simulink model "model1"  (Simulink 7.6)
settings: Solver=FixedStepDiscrete  StartTime=0.0  StopTime=10  FixedStep=1  RelTol=1e-3
libraries: simulink x6
settings Model: Creator=jordan  LastModifiedBy=jordan
settings OptimizationCC: BlockReduction=off  ConditionallyExecuteInputs=off

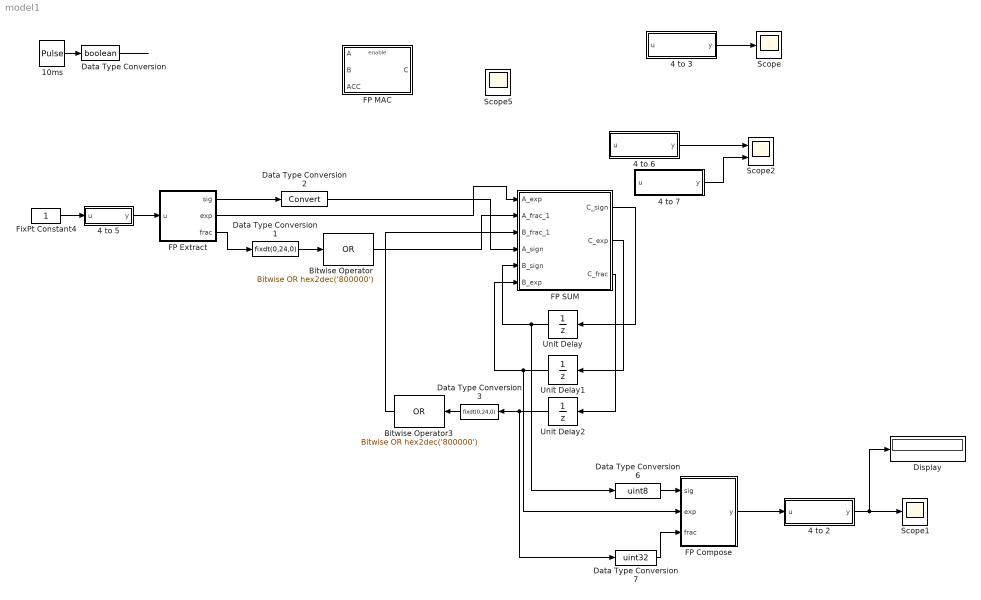
== system model1 ==
  10ms : DiscretePulseGenerator  Period=100
  4 to 2 : Stateflow chart  TreatAsAtomicUnit=on
  4 to 3 : Stateflow chart  TreatAsAtomicUnit=on
  4 to 5 : Stateflow chart  TreatAsAtomicUnit=on
  4 to 6 : Stateflow chart  TreatAsAtomicUnit=on
  4 to 7 : Stateflow chart  TreatAsAtomicUnit=on
  Bitwise Operator : simulink/Logic and Bit Operations/Bitwise Operator  logicop=OR  UseBitMask=on  BitMask=hex2dec('800000')  BitMaskRealWorld=Stored Integer
  Bitwise Operator3 : simulink/Logic and Bit Operations/Bitwise Operator  logicop=OR  UseBitMask=on  BitMask=hex2dec('800000')  BitMaskRealWorld=Stored Integer
  Data Type Conversion : DataTypeConversion  OutDataTypeStr=boolean
  Data Type Conversion1 : DataTypeConversion  OutDataTypeStr=fixdt(0,24,0)  RndMeth=Nearest
  Data Type Conversion2 : DataTypeConversion  RndMeth=Nearest
  Data Type Conversion3 : DataTypeConversion  OutDataTypeStr=fixdt(0,24,0)  RndMeth=Nearest
  Data Type Conversion6 : DataTypeConversion  OutDataTypeStr=uint8  RndMeth=Nearest
  Data Type Conversion7 : DataTypeConversion  OutDataTypeStr=uint32  RndMeth=Nearest
  Display : Display
  FP Compose : Stateflow chart  TreatAsAtomicUnit=on
  FP Extract : Stateflow chart  TreatAsAtomicUnit=on
  FP MAC : Subsystem
  FP SUM : Subsystem
  FixPt Constant4 : Constant  DisableCoverage=on  OutDataTypeStr=single  LockScale=on
  Scope : Scope
      settings: TimeRange=20.20725388601036  YMin=0  YMax=100  MaxDataPoints=50000
  Scope1 : Scope
      settings: SaveName=ScopeData3  MaxDataPoints=50000
  Scope2 : Scope  NumInputPorts=2
      settings: YMin=-5~-5  YMax=5~5  SaveName=ScopeData4  MaxDataPoints=50000
  Scope5 : Scope
      settings: SaveName=ScopeData11  MaxDataPoints=50000
  Unit Delay : UnitDelay  SampleTime=-1
  Unit Delay1 : UnitDelay  SampleTime=-1
  Unit Delay2 : UnitDelay  SampleTime=-1
  wires:
  10ms/1 -> Data Type Conversion/1
  Data Type Conversion/1 -> ?
  4 to 2/1(y) -> Scope1/1, Display/1
  4 to 6/1(y) -> Scope2/1
  4 to 7/1(y) -> Scope2/2
  4 to 3/1(y) -> Scope/1
  FP SUM/1(C_sign) -> Unit Delay/1
  FP SUM/2(C_exp) -> Unit Delay1/1
  FP SUM/3(C_frac) -> Unit Delay2/1
  Unit Delay/1 -> FP SUM/5(B_sign), Data Type Conversion6/1
  Unit Delay1/1 -> FP SUM/6(B_exp), FP Compose/2(exp)
  Unit Delay2/1 -> Data Type Conversion3/1, Data Type Conversion7/1
  Data Type Conversion3/1 -> Bitwise Operator3/1
  Bitwise Operator3/1 -> FP SUM/3(B_frac_1)
  FP Extract/1(sig) -> Data Type Conversion2/1
  FP Extract/2(exp) -> FP SUM/1(A_exp)
  Data Type Conversion1/1 -> Bitwise Operator/1
  FP Extract/3(frac) -> Data Type Conversion1/1
  Bitwise Operator/1 -> FP SUM/2(A_frac_1)
  Data Type Conversion6/1 -> FP Compose/1(sig)
  Data Type Conversion7/1 -> FP Compose/3(frac)
  FP Compose/1(y) -> 4 to 2/1(u)
  FixPt Constant4/1 -> 4 to 5/1(u)
  4 to 5/1(y) -> FP Extract/1(u)
  Data Type Conversion2/1 -> FP SUM/4(A_sign)

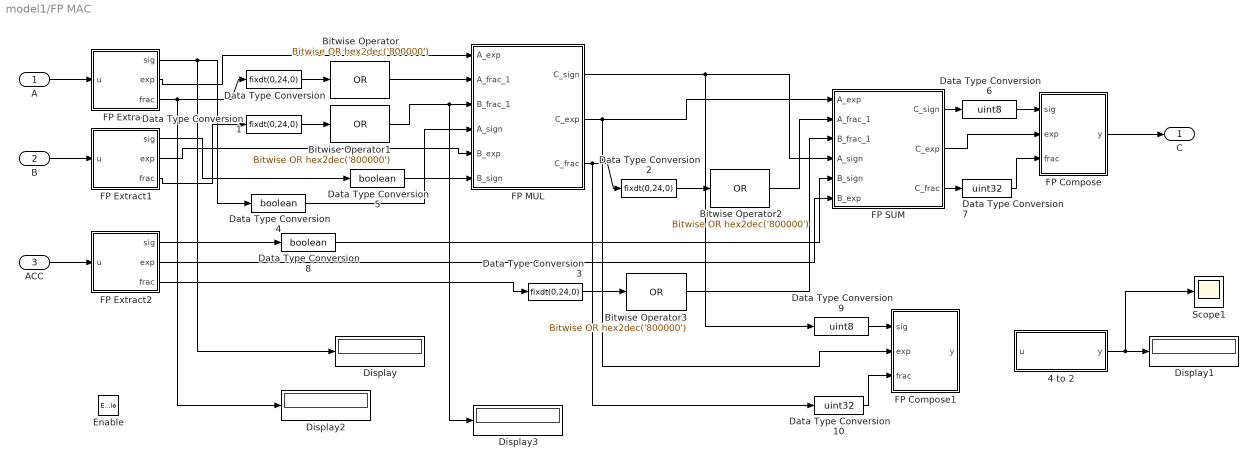
== system model1/FP MAC ==
  A : Inport
  B : Inport  Port=2
  ACC : Inport  Port=3
  Enable : EnablePort
  4 to 2 : Stateflow chart  TreatAsAtomicUnit=on
  Bitwise Operator{,1..3} (4 alike) : simulink/Logic and Bit Operations/Bitwise Operator  logicop=OR  UseBitMask=on  BitMask=hex2dec('800000')  BitMaskRealWorld=Stored Integer
  Data Type Conversion{,1..3} (4 alike) : DataTypeConversion  OutDataTypeStr=fixdt(0,24,0)  RndMeth=Nearest
  Data Type Conversion10 : DataTypeConversion  OutDataTypeStr=uint32  RndMeth=Nearest
  Data Type Conversion4 : DataTypeConversion  OutDataTypeStr=boolean  RndMeth=Nearest
  Data Type Conversion5 : DataTypeConversion  OutDataTypeStr=boolean  RndMeth=Nearest
  Data Type Conversion6 : DataTypeConversion  OutDataTypeStr=uint8  RndMeth=Nearest
  Data Type Conversion7 : DataTypeConversion  OutDataTypeStr=uint32  RndMeth=Nearest
  Data Type Conversion8 : DataTypeConversion  OutDataTypeStr=boolean  RndMeth=Nearest
  Data Type Conversion9 : DataTypeConversion  OutDataTypeStr=uint8  RndMeth=Nearest
  Display{,1..3} (4 alike) : Display
      Display3 settings: Format=hex (Stored Integer)
  FP Compose : Stateflow chart  TreatAsAtomicUnit=on
  FP Compose1 : Stateflow chart  TreatAsAtomicUnit=on
  FP Extract : Stateflow chart  TreatAsAtomicUnit=on
  FP Extract1 : Stateflow chart  TreatAsAtomicUnit=on
  FP Extract2 : Stateflow chart  TreatAsAtomicUnit=on
  FP MUL : Subsystem
  FP SUM : Subsystem
  Scope1 : Scope
      settings: SaveName=ScopeData9  MaxDataPoints=50000
  C : Outport  InitialOutput=0
  wires:
  A/1 -> FP Extract/1(u)
  B/1 -> FP Extract1/1(u)
  ACC/1 -> FP Extract2/1(u)
  FP Extract/1(sig) -> Data Type Conversion4/1, Display/1
  FP Extract1/1(sig) -> Data Type Conversion5/1
  FP Extract/2(exp) -> FP MUL/1(A_exp)
  FP Extract1/2(exp) -> FP MUL/5(B_exp)
  FP Extract/3(frac) -> Data Type Conversion/1, Display2/1
  FP Extract1/3(frac) -> Data Type Conversion1/1
  Data Type Conversion/1 -> Bitwise Operator/1
  Bitwise Operator/1 -> FP MUL/2(A_frac_1)
  Data Type Conversion1/1 -> Bitwise Operator1/1
  Bitwise Operator1/1 -> FP MUL/3(B_frac_1), Display3/1
  FP MUL/1(C_sign) -> FP SUM/4(A_sign), Data Type Conversion9/1
  FP MUL/2(C_exp) -> FP SUM/1(A_exp), FP Compose1/2(exp)
  FP MUL/3(C_frac) -> Data Type Conversion2/1, Data Type Conversion10/1
  Data Type Conversion2/1 -> Bitwise Operator2/1
  Bitwise Operator2/1 -> FP SUM/2(A_frac_1)
  FP Extract2/1(sig) -> Data Type Conversion8/1
  FP Extract2/2(exp) -> FP SUM/6(B_exp)
  FP Extract2/3(frac) -> Data Type Conversion3/1
  Data Type Conversion3/1 -> Bitwise Operator3/1
  Bitwise Operator3/1 -> FP SUM/3(B_frac_1)
  Data Type Conversion4/1 -> FP MUL/4(A_sign)
  Data Type Conversion5/1 -> FP MUL/6(B_sign)
  FP SUM/1(C_sign) -> Data Type Conversion6/1
  FP SUM/2(C_exp) -> FP Compose/2(exp)
  FP SUM/3(C_frac) -> Data Type Conversion7/1
  FP Compose/1(y) -> C/1
  Data Type Conversion6/1 -> FP Compose/1(sig)
  Data Type Conversion7/1 -> FP Compose/3(frac)
  Data Type Conversion8/1 -> FP SUM/5(B_sign)
  Data Type Conversion9/1 -> FP Compose1/1(sig)
  Data Type Conversion10/1 -> FP Compose1/3(frac)
  4 to 2/1(y) -> Display1/1, Scope1/1

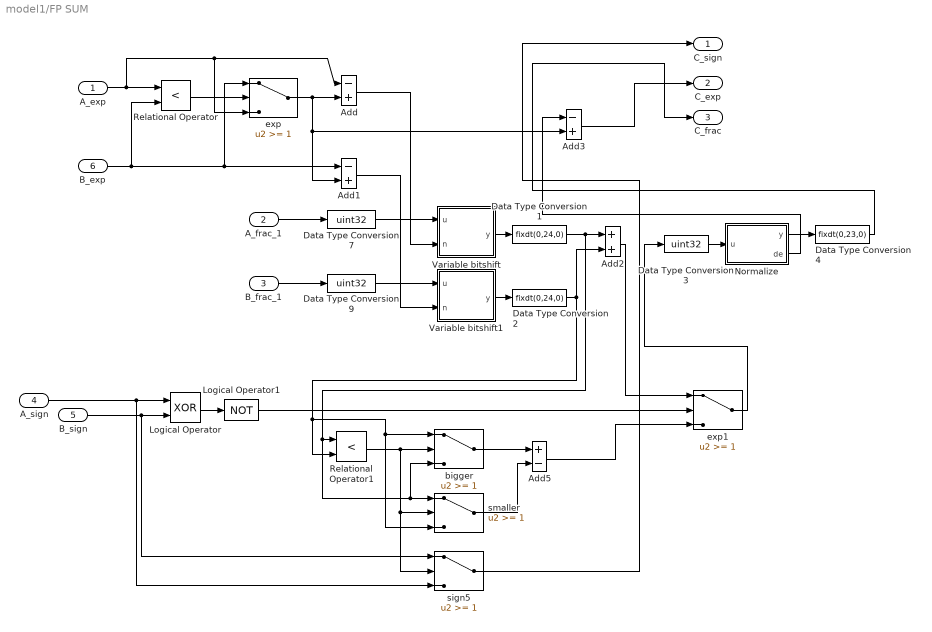
== system model1/FP SUM ==
  A_exp : Inport  OutDataTypeStr=uint8
  A_frac_1 : Inport  Port=2  OutDataTypeStr=fixdt(0,24,0)
  B_frac_1 : Inport  Port=3  OutDataTypeStr=fixdt(0,24,0)
  A_sign : Inport  Port=4  OutDataTypeStr=boolean
  B_sign : Inport  Port=5  OutDataTypeStr=boolean
  B_exp : Inport  Port=6  OutDataTypeStr=uint8
  Add : Sum  Inputs=-+  OutDataTypeStr=int8
  Add1 : Sum  Inputs=-+  OutDataTypeStr=int8
  Add2 : Sum  OutDataTypeStr=fixdt(0,25,0)  RndMeth=Nearest
  Add3 : Sum  Inputs=-+  OutDataTypeStr=uint8  SaturateOnIntegerOverflow=on
  Add5 : Sum  Inputs=+-  OutDataTypeStr=fixdt(0,25,0)  RndMeth=Nearest
  Data Type Conversion1 : DataTypeConversion  OutDataTypeStr=fixdt(0,24,0)
  Data Type Conversion2 : DataTypeConversion  OutDataTypeStr=fixdt(0,24,0)
  Data Type Conversion3 : DataTypeConversion  OutDataTypeStr=uint32
  Data Type Conversion4 : DataTypeConversion  OutDataTypeStr=fixdt(0,23,0)
  Data Type Conversion7 : DataTypeConversion  OutDataTypeStr=uint32
  Data Type Conversion9 : DataTypeConversion  OutDataTypeStr=uint32
  Logical Operator : Logic  Operator=XOR  AllPortsSameDT=off  OutDataTypeStr=boolean
  Logical Operator1 : Logic  Operator=NOT  AllPortsSameDT=off  OutDataTypeStr=boolean
  Normalize : Stateflow chart  TreatAsAtomicUnit=on
  Relational Operator : RelationalOperator  Operator=<  OutDataTypeStr=boolean
  Relational Operator1 : RelationalOperator  Operator=<  OutDataTypeStr=boolean
  Variable bitshift : Stateflow chart  TreatAsAtomicUnit=on
  Variable bitshift1 : Stateflow chart  TreatAsAtomicUnit=on
  bigger : Switch  Threshold=1
  exp : Switch  Threshold=1
  exp1 : Switch  Threshold=1
  sign5 : Switch  Threshold=1
  smaller : Switch  Threshold=1
  C_sign : Outport  OutDataTypeStr=boolean
  C_exp : Outport  Port=2  OutDataTypeStr=uint8
  C_frac : Outport  Port=3  OutDataTypeStr=fixdt(0,23,0)
  wires:
  Add3/1 -> C_exp/1
  B_sign/1 -> sign5/1, Logical Operator/2
  A_sign/1 -> sign5/3, Logical Operator/1
  Data Type Conversion9/1 -> Variable bitshift1/1(u)
  Data Type Conversion7/1 -> Variable bitshift/1(u)
  sign5/1 -> C_sign/1
  exp1/1 -> Data Type Conversion3/1
  Add5/1 -> exp1/3
  smaller/1 -> Add5/2
  bigger/1 -> Add5/1
  Relational Operator1/1 -> sign5/2, smaller/2, bigger/2
  Logical Operator1/1 -> exp1/2
  Logical Operator/1 -> Logical Operator1/1
  Data Type Conversion4/1 -> C_frac/1
  Data Type Conversion3/1 -> Normalize/1(u)
  Normalize/2(de) -> Add3/1
  Normalize/1(y) -> Data Type Conversion4/1
  Add2/1 -> exp1/1
  Data Type Conversion2/1 -> smaller/3, bigger/1, Relational Operator1/2, Add2/2
  Variable bitshift1/1(y) -> Data Type Conversion2/1
  Add1/1 -> Variable bitshift1/2(n)
  Add/1 -> Variable bitshift/2(n)
  B_frac_1/1 -> Data Type Conversion9/1
  exp/1 -> Add3/2, Add1/2, Add/2
  Relational Operator/1 -> exp/2
  Data Type Conversion1/1 -> bigger/3, smaller/1, Relational Operator1/1, Add2/1
  Variable bitshift/1(y) -> Data Type Conversion1/1
  A_frac_1/1 -> Data Type Conversion7/1
  B_exp/1 -> Relational Operator/2, Add1/1, exp/1
  A_exp/1 -> Add/1, exp/3, Relational Operator/1

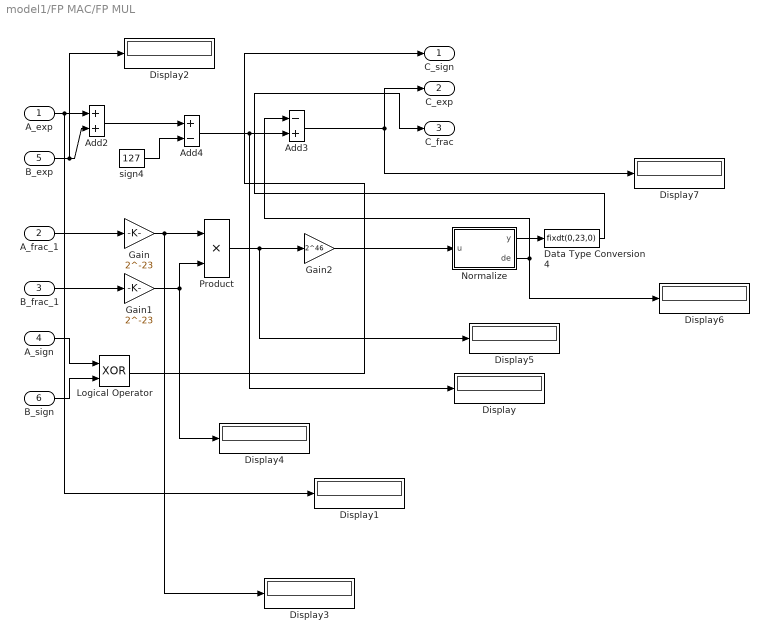
== system model1/FP MAC/FP MUL ==
  A_exp : Inport  OutDataTypeStr=uint8
  A_frac_1 : Inport  Port=2  OutDataTypeStr=fixdt(0,24,0)
  B_frac_1 : Inport  Port=3  OutDataTypeStr=fixdt(0,24,0)
  A_sign : Inport  Port=4  OutDataTypeStr=boolean
  B_exp : Inport  Port=5  OutDataTypeStr=uint8
  B_sign : Inport  Port=6  OutDataTypeStr=boolean
  Add2 : Sum  OutDataTypeStr=fixdt(0,9,0)  RndMeth=Nearest
  Add3 : Sum  Inputs=-+  OutDataTypeStr=uint8  RndMeth=Nearest  SaturateOnIntegerOverflow=on
  Add4 : Sum  Inputs=+-  OutDataTypeStr=uint8  RndMeth=Nearest  SaturateOnIntegerOverflow=on
  Data Type Conversion4 : DataTypeConversion  OutDataTypeStr=fixdt(0,23,0)
  Display{,1..7} (8 alike) : Display
  Gain : Gain  Gain=2^-23  OutDataTypeStr=fixdt(0,24,23)  RndMeth=Nearest
  Gain1 : Gain  Gain=2^-23  OutDataTypeStr=fixdt(0,24,23)  RndMeth=Nearest
  Gain2 : Gain  Gain=2^46  OutDataTypeStr=fixdt(0,48,0)  RndMeth=Nearest
  Logical Operator : Logic  Operator=XOR  AllPortsSameDT=off  OutDataTypeStr=boolean
  Normalize : Stateflow chart  TreatAsAtomicUnit=on
  Product : Product  OutDataTypeStr=fixdt(0,48,46)  RndMeth=Nearest
  sign4 : Constant  Value=127  OutDataTypeStr=fixdt(0,9,0)
  C_sign : Outport  OutDataTypeStr=boolean
  C_exp : Outport  Port=2  OutDataTypeStr=uint8
  C_frac : Outport  Port=3  OutDataTypeStr=fixdt(0,23,0)
  wires:
  B_exp/1 -> Add2/2, Display2/1
  Normalize/1(y) -> Data Type Conversion4/1
  Normalize/2(de) -> Add3/1, Display6/1
  Add3/1 -> C_exp/1, Display7/1
  Data Type Conversion4/1 -> C_frac/1
  Logical Operator/1 -> C_sign/1
  Product/1 -> Display5/1, Gain2/1
  Add2/1 -> Add4/1
  sign4/1 -> Add4/2
  Add4/1 -> Add3/2, Display/1
  Gain/1 -> Product/1, Display3/1
  Gain1/1 -> Product/2, Display4/1
  A_frac_1/1 -> Gain/1
  B_frac_1/1 -> Gain1/1
  A_sign/1 -> Logical Operator/1
  A_exp/1 -> Add2/1, Display1/1
  B_sign/1 -> Logical Operator/2
  Gain2/1 -> Normalize/1(u)

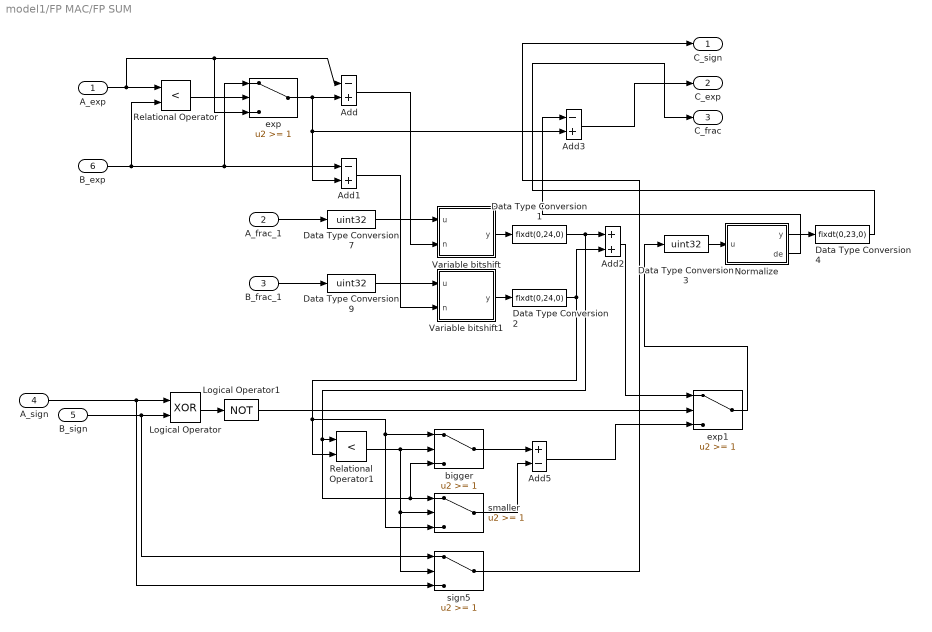
== system model1/FP MAC/FP SUM ==
  A_exp : Inport  OutDataTypeStr=uint8
  A_frac_1 : Inport  Port=2  OutDataTypeStr=fixdt(0,24,0)
  B_frac_1 : Inport  Port=3  OutDataTypeStr=fixdt(0,24,0)
  A_sign : Inport  Port=4  OutDataTypeStr=boolean
  B_sign : Inport  Port=5  OutDataTypeStr=boolean
  B_exp : Inport  Port=6  OutDataTypeStr=uint8
  Add : Sum  Inputs=-+  OutDataTypeStr=int8
  Add1 : Sum  Inputs=-+  OutDataTypeStr=int8
  Add2 : Sum  OutDataTypeStr=fixdt(0,25,0)  RndMeth=Nearest
  Add3 : Sum  Inputs=-+  OutDataTypeStr=uint8  SaturateOnIntegerOverflow=on
  Add5 : Sum  Inputs=+-  OutDataTypeStr=fixdt(0,25,0)  RndMeth=Nearest
  Data Type Conversion1 : DataTypeConversion  OutDataTypeStr=fixdt(0,24,0)
  Data Type Conversion2 : DataTypeConversion  OutDataTypeStr=fixdt(0,24,0)
  Data Type Conversion3 : DataTypeConversion  OutDataTypeStr=uint32
  Data Type Conversion4 : DataTypeConversion  OutDataTypeStr=fixdt(0,23,0)
  Data Type Conversion7 : DataTypeConversion  OutDataTypeStr=uint32
  Data Type Conversion9 : DataTypeConversion  OutDataTypeStr=uint32
  Logical Operator : Logic  Operator=XOR  AllPortsSameDT=off  OutDataTypeStr=boolean
  Logical Operator1 : Logic  Operator=NOT  AllPortsSameDT=off  OutDataTypeStr=boolean
  Normalize : Stateflow chart  TreatAsAtomicUnit=on
  Relational Operator : RelationalOperator  Operator=<  OutDataTypeStr=boolean
  Relational Operator1 : RelationalOperator  Operator=<  OutDataTypeStr=boolean
  Variable bitshift : Stateflow chart  TreatAsAtomicUnit=on
  Variable bitshift1 : Stateflow chart  TreatAsAtomicUnit=on
  bigger : Switch  Threshold=1
  exp : Switch  Threshold=1
  exp1 : Switch  Threshold=1
  sign5 : Switch  Threshold=1
  smaller : Switch  Threshold=1
  C_sign : Outport  OutDataTypeStr=boolean
  C_exp : Outport  Port=2  OutDataTypeStr=uint8
  C_frac : Outport  Port=3  OutDataTypeStr=fixdt(0,23,0)
  wires:
  A_exp/1 -> Relational Operator/1, exp/3, Add/1
  B_exp/1 -> exp/1, Add1/1, Relational Operator/2
  A_frac_1/1 -> Data Type Conversion7/1
  Variable bitshift/1(y) -> Data Type Conversion1/1
  Data Type Conversion1/1 -> Add2/1, Relational Operator1/1, smaller/1, bigger/3
  Relational Operator/1 -> exp/2
  exp/1 -> Add/2, Add1/2, Add3/2
  B_frac_1/1 -> Data Type Conversion9/1
  Add/1 -> Variable bitshift/2(n)
  Add1/1 -> Variable bitshift1/2(n)
  Variable bitshift1/1(y) -> Data Type Conversion2/1
  Data Type Conversion2/1 -> Add2/2, Relational Operator1/2, bigger/1, smaller/3
  Add2/1 -> exp1/1
  Normalize/1(y) -> Data Type Conversion4/1
  Normalize/2(de) -> Add3/1
  Data Type Conversion3/1 -> Normalize/1(u)
  Data Type Conversion4/1 -> C_frac/1
  Logical Operator/1 -> Logical Operator1/1
  Logical Operator1/1 -> exp1/2
  Relational Operator1/1 -> bigger/2, smaller/2, sign5/2
  bigger/1 -> Add5/1
  smaller/1 -> Add5/2
  Add5/1 -> exp1/3
  exp1/1 -> Data Type Conversion3/1
  sign5/1 -> C_sign/1
  Data Type Conversion7/1 -> Variable bitshift/1(u)
  Data Type Conversion9/1 -> Variable bitshift1/1(u)
  A_sign/1 -> Logical Operator/1, sign5/3
  B_sign/1 -> Logical Operator/2, sign5/1
  Add3/1 -> C_exp/1

== matlab function FP SUM/Normalize ==
  data: u input uint32; y output uint32; de output double
function [y,de] = fcn(u)
%#eml

buf=u;
p=int8(-1);
c=bitand(buf,2^24);
for ind=1:25
    if (~c)
        p=p+1;
        buf=bitshift(buf,1);
        c=bitand(buf,2^24);
    end
end
bufy = bitand(bitshift(u,p),2^23-1);
y=bufy;
de=p;

== matlab function FP SUM/Variable bitshift ==
  data: u input uint32; y output uint32; n input int8
function y = fcn(u,n)
%#eml

y = bitshift(u,-n);

== matlab function FP MAC/FP SUM/Normalize ==
  data: u input uint32; y output uint32; de output double
function [y,de] = fcn(u)
%#eml

buf=u;
p=int8(-1);
c=bitand(buf,2^24);
for ind=1:25
    if (~c)
        p=p+1;
        buf=bitshift(buf,1);
        c=bitand(buf,2^24);
    end
end
bufy = bitand(bitshift(u,p),2^23-1);
y=bufy;
de=p;

== matlab function 4 to 3 ==
  data: y output single; u input uint32
function y  = fcn(u)
%#eml
y=typecast(u,'single');

== matlab function FP MAC/FP SUM/Variable bitshift ==
  data: u input uint32; y output uint32; n input int8
function y = fcn(u,n)
%#eml

y = bitshift(u,-n);

== matlab function FP SUM/Variable bitshift1 ==
  data: u input uint32; y output uint32; n input int8
function y = fcn(u,n)
%#eml

y = bitshift(u,-n);

== matlab function FP MAC/FP SUM/Variable bitshift1 ==
  data: u input uint32; y output uint32; n input int8
function y = fcn(u,n)
%#eml

y = bitshift(u,-n);

== matlab function FP Extract ==
  data: u input uint32; sig output uint8; exp output uint8; frac output uint32
function [sig,exp,frac] = fcn(u)
%#eml

z=u;
sig=uint8(bitshift(z,-31));
exp=uint8(bitshift(bitshift(z,1),-24));
frac=uint32(bitand(z,8388607));
%bexp=uint8(bitshift(bitshift(z,1),-23));
% exp1=uint8(zeros(8,1));
% frac1=uint8(zeros(23,1));
% for ind=0:7
%     exp1(ind+1)=uint8(bitand(bitshift(bexp,-ind),1));
% end
% bfrac=z;
% for ind=0:22
%     frac1(ind+1)=uint8(bitand(bitshift(bfrac,-ind),1));
% end
% exp=exp1;
% frac=frac1;

== matlab function FP MAC/FP MUL/Normalize ==
  data: u input fixdt(0,48,0); y output uint32; de output double
function [y,de] = fcn(u)
%#eml

buf=u;
p=int8(-1);
c=bitand(buf,fi(2^47,0,48,0));
for ind=1:25
    if (c==0)
        p=p+1;
        buf=bitshift(buf,1);
        c=bitand(buf,fi(2^47,0,48,0));
    end
end
bufy = bitand(bitshift(u,p),fi(2^46-1,0,48,0));
y=uint32(bitshift(bufy,-23));
de=p;

== matlab function FP Compose ==
  data: sig input uint8; exp input uint8; frac input uint32; y output uint32
function y = fcn(sig,exp,frac)
%#eml

z=uint32(0);
if sig
    z=uint32(bitshift(uint32(1),31));
end
buf=uint32(bitshift(uint32(exp),23));
z=bitor(z,buf);
z=bitor(z,frac);
y=z;

== matlab function FP MAC/FP Extract ==
  data: u input uint32; sig output uint8; exp output uint8; frac output uint32
function [sig,exp,frac] = fcn(u)
%#eml

z=u;
sig=uint8(bitshift(z,-31));
exp=uint8(bitshift(bitshift(z,1),-24));
frac=uint32(bitand(z,8388607));
%bexp=uint8(bitshift(bitshift(z,1),-23));
% exp1=uint8(zeros(8,1));
% frac1=uint8(zeros(23,1));
% for ind=0:7
%     exp1(ind+1)=uint8(bitand(bitshift(bexp,-ind),1));
% end
% bfrac=z;
% for ind=0:22
%     frac1(ind+1)=uint8(bitand(bitshift(bfrac,-ind),1));
% end
% exp=exp1;
% frac=frac1;

== matlab function FP MAC/FP Extract1 ==
  data: u input uint32; sig output uint8; exp output uint8; frac output uint32
function [sig,exp,frac] = fcn(u)
%#eml

z=u;
sig=uint8(bitshift(z,-31));
exp=uint8(bitshift(bitshift(z,1),-24));
frac=uint32(bitand(z,8388607));
%bexp=uint8(bitshift(bitshift(z,1),-23));
% exp1=uint8(zeros(8,1));
% frac1=uint8(zeros(23,1));
% for ind=0:7
%     exp1(ind+1)=uint8(bitand(bitshift(bexp,-ind),1));
% end
% bfrac=z;
% for ind=0:22
%     frac1(ind+1)=uint8(bitand(bitshift(bfrac,-ind),1));
% end
% exp=exp1;
% frac=frac1;

== matlab function FP MAC/FP Extract2 ==
  data: u input uint32; sig output uint8; exp output uint8; frac output uint32
function [sig,exp,frac] = fcn(u)
%#eml

z=u;
sig=uint8(bitshift(z,-31));
exp=uint8(bitshift(bitshift(z,1),-24));
frac=uint32(bitand(z,8388607));
%bexp=uint8(bitshift(bitshift(z,1),-23));
% exp1=uint8(zeros(8,1));
% frac1=uint8(zeros(23,1));
% for ind=0:7
%     exp1(ind+1)=uint8(bitand(bitshift(bexp,-ind),1));
% end
% bfrac=z;
% for ind=0:22
%     frac1(ind+1)=uint8(bitand(bitshift(bfrac,-ind),1));
% end
% exp=exp1;
% frac=frac1;

== matlab function FP MAC/FP Compose ==
  data: sig input uint8; exp input uint8; frac input uint32; y output uint32
function y = fcn(sig,exp,frac)
%#eml

z=uint32(0);
if sig
    z=uint32(bitshift(uint32(1),31));
end
buf=uint32(bitshift(uint32(exp),23));
z=bitor(z,buf);
z=bitor(z,frac);
y=z;

== matlab function 4 to 2 ==
  data: y output single; u input uint32
function y  = fcn(u)
%#eml
y=typecast(u,'single');

== matlab function 4 to 5 ==
  data: y output uint32; u input single
function y  = fcn(u)
%#eml
y=typecast(u,'uint32');

== matlab function FP MAC/4 to 2 ==
  data: y output single; u input uint32
function y  = fcn(u)
%#eml
y=typecast(u,'single');

== matlab function FP MAC/FP Compose1 ==
  data: sig input uint8; exp input uint8; frac input uint32; y output uint32
function y = fcn(sig,exp,frac)
%#eml

z=uint32(0);
if sig
    z=uint32(bitshift(uint32(1),31));
end
buf=uint32(bitshift(uint32(exp),23));
z=bitor(z,buf);
z=bitor(z,frac);
y=z;

== matlab function 4 to 6 ==
  data: y output single; u input uint32
function y  = fcn(u)
%#eml
y=typecast(u,'single');

== matlab function 4 to 7 ==
  data: y output single; u input uint32
function y  = fcn(u)
%#eml
y=typecast(u,'single');
